simulink model "schema"  (Simulink 7.4)
settings: Solver=ode45  StartTime=0.0  StopTime=10.0  RelTol=1e-3
libraries: simulink x1
settings Model: Creator=a.pajxaev.2018  LastModifiedBy=a.pajxaev.2018

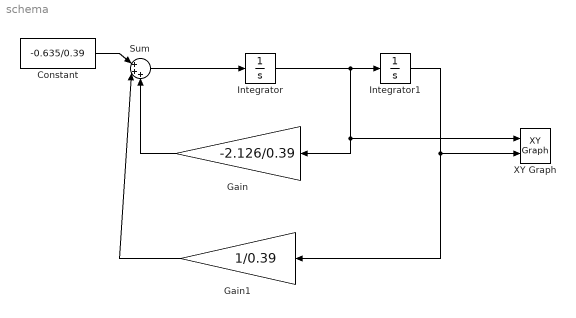
== system schema ==
  Constant : Constant  Value=-0.635/0.39  OutDataType=fixdt(1, 16)  OutScaling=2^0
  Gain : Gain  Gain=-2.126/0.39  ParameterDataType=fixdt(1, 16)  ParameterScaling=2^0  OutDataType=fixdt(1, 16)  OutScaling=2^0
  Gain1 : Gain  Gain=1/0.39  ParameterDataType=fixdt(1, 16)  ParameterScaling=2^0  OutDataType=fixdt(1, 16)  OutScaling=2^0
  Integrator : Integrator  InitialCondition=0.2
  Integrator1 : Integrator  InitialCondition=-0.2
  Sum : Sum  Inputs=|+++  OutDataType=fixdt(1, 16)  OutScaling=2^0
  XY Graph : simulink/Sinks/XY Graph  SystemSampleTime=-1  xmin=-1  xmax=1  ymin=-1  ymax=1  st=-1
  wires:
  Constant/1 -> Sum/1
  Sum/1 -> Integrator/1
  Integrator/1 -> Integrator1/1, Gain/1, XY Graph/1
  Gain/1 -> Sum/3
  Integrator1/1 -> Gain1/1, XY Graph/2
  Gain1/1 -> Sum/2
